simulink model "MGcircuit"  (R2020b)
settings: Solver=VariableStepAuto  StartTime=0.0  StopTime=10  FixedStep=0.0002  RelTol=1e-3
libraries: fl_lib x44, nesl_utility x3, ee_lib x3
settings Model: Creator=tian  LastModifiedBy=tian
settings SolverCC: ZeroCrossAlgorithm=Adaptive
settings DebuggingCC: IgnoredZcDiagnostic=none

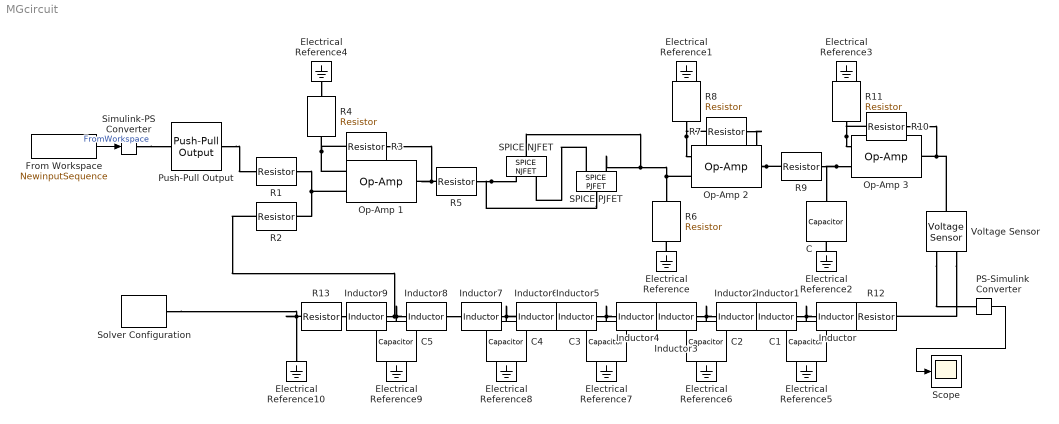
== system MGcircuit ==
  C : fl_lib/Electrical/Electrical Elements/Capacitor  c=100 nF  r=1e-6 Ohm  g=0 1/Ohm  i_specify=off  i_priority=None  i=0 A  i_nominal_specify=off  i_nominal_unit=A  i_nominal_value=1  v_specify=on  v_priority=None  v=2 V  v_nominal_specify=off  v_nominal_unit=V  v_nominal_value=1  vc_specify=off  vc_priority=High  vc=0 V  vc_nominal_specify=off  vc_nominal_unit=V  vc_nominal_value=1
  C{1..5} (5 alike) : fl_lib/Electrical/Electrical Elements/Capacitor  c=525 nF  r=1e-6 Ohm  g=0 1/Ohm  i_specify=off  i_priority=None  i=0 A  i_nominal_specify=off  i_nominal_unit=A  i_nominal_value=1  v_specify=off  v_priority=None  v=0 V  v_nominal_specify=off  v_nominal_unit=V  v_nominal_value=1  vc_specify=off  vc_priority=High  vc=0 V  vc_nominal_specify=off  vc_nominal_unit=V  vc_nominal_value=1
  Electrical Reference{,1..10} (11 alike) : fl_lib/Electrical/Electrical Elements/Electrical Reference
  From Workspace : FromWorkspace  VariableName=NewinputSequence
  Inductor{,1..9} (10 alike) : fl_lib/Electrical/Electrical Elements/Inductor  l=9.5 mH  r=0 Ohm  g=1e-9 1/Ohm  i_specify=off  i_priority=None  i=0 A  i_nominal_specify=off  i_nominal_unit=A  i_nominal_value=1  v_specify=off  v_priority=None  v=0 V  v_nominal_specify=off  v_nominal_unit=V  v_nominal_value=1  i_L_specify=off  i_L_priority=High  i_L=0 A  i_L_nominal_specify=off  i_L_nominal_unit=A  i_L_nominal_value=1
  Op-Amp 1 : fl_lib/Electrical/Electrical Elements/Op-Amp  outI_specify=off  outI_priority=None  outI=0 A  outI_nominal_specify=off  outI_nominal_unit=A  outI_nominal_value=1
  Op-Amp 2 : fl_lib/Electrical/Electrical Elements/Op-Amp  outI_specify=off  outI_priority=None  outI=0 A  outI_nominal_specify=off  outI_nominal_unit=A  outI_nominal_value=1
  Op-Amp 3 : fl_lib/Electrical/Electrical Elements/Op-Amp  outI_specify=off  outI_priority=None  outI=0 A  outI_nominal_specify=off  outI_nominal_unit=A  outI_nominal_value=1
  PS-Simulink Converter : nesl_utility/PS-Simulink Converter  PhysicalDomain=network_engine_domain  SubClassName=ps_output  LeftPortType=input  RightPortType=output  PseudoPeriodic=off  Frequencies=[]  Unit=inherit  AffineConversion=off
  Push-Pull Output : ee_lib/Integrated Circuits/Push-Pull Output  k=1 V  c=0  output_type=1  V_neg=0 V  V_pos=5 V  V_meas=[0, 5] V  R_OUT=25 Ohm  R_OH=[25, 250] Ohm  I_OH=63 mA  R_OL=[30, 800] Ohm  I_OL=-45 mA  Delay=25 ns  Ron=5 Ohm  Vf=0.6 V  V0=0.01 V  X0=0
      settings: SourceProductBaseCode=PS  InternalSimscapePortConfiguration="{\"Bottom\":[],\"Left\":[{\"id\":\"X\",\"label\":\"X\",\"type\":\"input\"}],\"Right\":[{\"id\":\"J\",\"label\":\"\",\"type\":\"foundation.electrical.electrical\"}],\"Top\":[]}"
  R1 : fl_lib/Electrical/Electrical Elements/Resistor  R=1 kOhm  i_specify=off  i_priority=None  i=0 A  i_nominal_specify=off  i_nominal_unit=A  i_nominal_value=1  v_specify=off  v_priority=None  v=0 V  v_nominal_specify=off  v_nominal_unit=V  v_nominal_value=1
  R{3..4,9..11} (5 alike) : fl_lib/Electrical/Electrical Elements/Resistor  R=3 kOhm  i_specify=off  i_priority=None  i=0 A  i_nominal_specify=off  i_nominal_unit=A  i_nominal_value=1  v_specify=off  v_priority=None  v=0 V  v_nominal_specify=off  v_nominal_unit=V  v_nominal_value=1
  R12 : fl_lib/Electrical/Electrical Elements/Resistor  R=135 Ohm  i_specify=off  i_priority=None  i=0 A  i_nominal_specify=off  i_nominal_unit=A  i_nominal_value=1  v_specify=off  v_priority=None  v=0 V  v_nominal_specify=off  v_nominal_unit=V  v_nominal_value=1
  R13 : fl_lib/Electrical/Electrical Elements/Resistor  R=135 Ohm  i_specify=off  i_priority=None  i=0 A  i_nominal_specify=off  i_nominal_unit=A  i_nominal_value=1  v_specify=off  v_priority=None  v=0 V  v_nominal_specify=off  v_nominal_unit=V  v_nominal_value=1
  R2 : fl_lib/Electrical/Electrical Elements/Resistor  R=1 kOhm  i_specify=off  i_priority=None  i=0 A  i_nominal_specify=off  i_nominal_unit=A  i_nominal_value=1  v_specify=off  v_priority=None  v=0 V  v_nominal_specify=off  v_nominal_unit=V  v_nominal_value=1
  R5 : fl_lib/Electrical/Electrical Elements/Resistor  R=100 Ohm  i_specify=off  i_priority=None  i=0 A  i_nominal_specify=off  i_nominal_unit=A  i_nominal_value=1  v_specify=off  v_priority=None  v=0 V  v_nominal_specify=off  v_nominal_unit=V  v_nominal_value=1
  R6 : fl_lib/Electrical/Electrical Elements/Resistor  R=560 Ohm  i_specify=off  i_priority=None  i=0 A  i_nominal_specify=off  i_nominal_unit=A  i_nominal_value=1  v_specify=off  v_priority=None  v=0 V  v_nominal_specify=off  v_nominal_unit=V  v_nominal_value=1
  R7 : fl_lib/Electrical/Electrical Elements/Resistor  R=4 kOhm  i_specify=off  i_priority=None  i=0 A  i_nominal_specify=off  i_nominal_unit=A  i_nominal_value=1  v_specify=off  v_priority=None  v=0 V  v_nominal_specify=off  v_nominal_unit=V  v_nominal_value=1
  R8 : fl_lib/Electrical/Electrical Elements/Resistor  R=1 kOhm  i_specify=off  i_priority=None  i=0 A  i_nominal_specify=off  i_nominal_unit=A  i_nominal_value=1  v_specify=off  v_priority=None  v=0 V  v_nominal_specify=off  v_nominal_unit=V  v_nominal_value=1
  SPICE NJFET : ee_lib/Additional Components/SPICE Semiconductors/SPICE NJFET  AREA=1.0 m^2  SCALE=1  VTO=-1.372 V  BETA=1.125e-3 A/m^2/V^2  LAMBDA=2.3e-3 1/V  IS=181.3e-15 A/m^2  RD=1 m^2*Ohm  RS=1 m^2*Ohm  N=1  C_param=2  CGS=4.62e-12 F/m^2  CGD=2.92e-12 F/m^2  VJ=1 V  M=0.5  FC=0.5  T_param=1  XTI=0  EG=1.11 eV  TFIXED=300.15 K  TMEAS=300.15 K  IC_given=1  ICVDS=0 V  ICVGS=0 V  TOFFSET=0 K
      settings: SourceProductBaseCode=PS  InternalSimscapePortConfiguration="{\"Bottom\":[],\"Left\":[{\"id\":\"gx\",\"label\":\"\",\"type\":\"foundation.electrical.electrical\"}],\"Right\":[{\"id\":\"dx\",\"label\":\"\",\"type\":\"foundation.electrical.electrical\"},{\"id\":\"sx\",\"label\":\"\",\"type\":\"foundation.electrical.electrical\"}],\"Top\":[]}"
  SPICE PJFET : ee_lib/Additional Components/SPICE Semiconductors/SPICE PJFET  AREA=1.0 m^2  SCALE=1  VTO=-1.75 V  BETA=1.107e-3 A/m^2/V^2  LAMBDA=20e-3 1/V  IS=222.4e-15 A/m^2  RD=1 m^2*Ohm  RS=1 m^2*Ohm  N=1  C_param=2  CGS=2.34e-12 F/m^2  CGD=2.92e-12 F/m^2  VJ=1 V  M=0.5  FC=0.5  T_param=1  XTI=0  EG=1.11 eV  TFIXED=300.15 K  TMEAS=300.15 K  IC_given=1  ICVDS=0 V  ICVGS=0 V  TOFFSET=0 K
      settings: SourceProductBaseCode=PS  InternalSimscapePortConfiguration="{\"Bottom\":[],\"Left\":[{\"id\":\"gx\",\"label\":\"\",\"type\":\"foundation.electrical.electrical\"}],\"Right\":[{\"id\":\"dx\",\"label\":\"\",\"type\":\"foundation.electrical.electrical\"},{\"id\":\"sx\",\"label\":\"\",\"type\":\"foundation.electrical.electrical\"}],\"Top\":[]}"
  Scope : Scope
  Simulink-PS Converter : nesl_utility/Simulink-PS Converter  PhysicalDomain=network_engine_domain  SubClassName=ps_input  LeftPortType=input  RightPortType=output  PseudoPeriodic=off  Frequencies=[]  NoiseDistribution=none  NoiseParameters=[]  Unit=1  AffineConversion=off  FilteringAndDerivatives=provide  SimscapeFilterOrder=1  InputFilterTimeConstant=0.001  UdotUserProvided=0
  Solver Configuration : nesl_utility/Solver Configuration  PhysicalDomain=network_engine_domain  SubClassName=solver  LeftPortType=input  RightPortType=generic  Tones=[]  Harmonics=[]  SimulateNoise=off  Profile=off  UseLocalSampling=off  EnableSwitchedLinearOptims=on  FrequencyDomain=off  UseCCode=off  RelTol=0.001  AbsTol=1e-06  MinStep=1e-09  ToWorkspace=off  RevertToSquareIcSolve=off  NumHomotopyIterations=100  PhasorMode=off  PhasorModeNumHarmonics=1  DoDC=off  ResidualTolerance=1e-09  UseLocalSolver=off  LocalSolverChoice=NE_BACKWARD_EULER_ADVANCER  LocalSolverSampleTime=0.001  DoFixedCost=off  MaxNonlinIter=3  MaxModeIter=2  ComputeImpulses=off  ImpulseIterations=2  LinearAlgebra=auto  EquationFormulation=NE_TIME_EF  DelaysMemoryBudget=1024  AutomaticFiltering=on  FilteringTimeConstant=0.001  PartitionStorageMethod=AS_NEEDED  PartitionMemoryBudget=1024  PartitionMethod=ROBUST
  Voltage Sensor : fl_lib/Electrical/Electrical Sensors/Voltage Sensor
  wires:
  PS-Simulink Converter/1 -> Scope/1
  From Workspace/1 -> Simulink-PS Converter/1  "FromWorkspace"
  connections:
  Op-Amp 2/LConn1 -- SPICE NJFET/LConn1 -- SPICE PJFET/RConn2 -- R6/LConn1
  Electrical Reference/LConn1 -- R6/RConn1
  R5/RConn1 -- SPICE PJFET/LConn1 -- SPICE NJFET/RConn2
  R8/LConn1 -- Op-Amp 2/LConn2 -- R7/LConn1
  R8/RConn1 -- Electrical Reference1/LConn1
  R9/LConn1 -- Op-Amp 2/RConn1 -- R7/RConn1
  R9/RConn1 -- C/LConn1 -- Op-Amp 3/LConn1
  Electrical Reference2/LConn1 -- C/RConn1
  R11/LConn1 -- R10/LConn1 -- Op-Amp 3/LConn2
  Electrical Reference3/LConn1 -- R11/RConn1
  R10/RConn1 -- Voltage Sensor/LConn1 -- Op-Amp 3/RConn1
  Op-Amp 1/LConn2 -- R3/LConn1 -- R4/LConn1
  Electrical Reference4/LConn1 -- R4/RConn1
  R1/RConn1 -- Op-Amp 1/LConn1 -- R2/RConn1
  Inductor/LConn1 -- R12/RConn1
  Inductor1/LConn1 -- Inductor/RConn1 -- C1/LConn1
  Inductor4/LConn1 -- Inductor3/RConn1
  Inductor5/LConn1 -- Inductor4/RConn1 -- C3/LConn1
  Inductor2/LConn1 -- Inductor1/RConn1
  Inductor3/LConn1 -- Inductor2/RConn1 -- C2/LConn1
  Inductor6/LConn1 -- Inductor5/RConn1
  Inductor7/LConn1 -- Inductor6/RConn1 -- C4/LConn1
  Inductor8/LConn1 -- Inductor7/RConn1
  Inductor9/LConn1 -- Inductor8/RConn1 -- R2/LConn1 -- C5/LConn1
  Electrical Reference5/LConn1 -- C1/RConn1
  Electrical Reference6/LConn1 -- C2/RConn1
  Electrical Reference7/LConn1 -- C3/RConn1
  Electrical Reference8/LConn1 -- C4/RConn1
  Electrical Reference9/LConn1 -- C5/RConn1
  R13/LConn1 -- Inductor9/RConn1
  R13/RConn1 -- Electrical Reference10/LConn1 -- Solver Configuration/RConn1
  SPICE PJFET/RConn1 -- SPICE NJFET/RConn1
  Voltage Sensor/RConn1 -- PS-Simulink Converter/LConn1
  Voltage Sensor/RConn2 -- R12/LConn1
  Simulink-PS Converter/RConn1 -- Push-Pull Output/LConn1
  Push-Pull Output/RConn1 -- R1/LConn1
  R3/RConn1 -- R5/LConn1 -- Op-Amp 1/RConn1
